simulink model "mpc_model_control_robot_with_forces"  (Simulink 8.0)
settings: Solver=ode3  StartTime=0.0  StopTime=delta_t  FixedStep=0.0002  RelTol=1e-3
values from neighbouring files (symbols this model uses):
  all_J_T_K_J = all_J_T_K_J + J_cont'*K_cont*J_cont    [run_control_tests_no_obstacles_testing_model_prediction.m]    (also in run_control_tests_with_force.m; run_control_tests_with_force_and_model_prediction.m; run_control_tests_with_force_kreacher.m; run_control_tests_with_force_vary_stiffness_and_delta_t.m)
  all_J_T_Kd_J = all_J_T_Kd_J + J_cont'*Kd_cont*J_cont    [run_control_tests_no_obstacles_testing_model_prediction.m]    (also in run_control_tests_with_force.m; run_control_tests_with_force_and_model_prediction.m; run_control_tests_with_force_vary_stiffness_and_delta_t.m; run_control_tests_with_obstacles_testing_model_prediction.m)
  Kd = diag([kd, kd, kd, kd])    [run_control_tests_no_force_vary_time_horizon_kreacher.m]    (also in run_control_tests_no_force_vary_time_horizon_kreacher_QS.m; run_control_tests_no_force_vary_time_horizon_single_link.m = diag([kd]); run_control_tests_no_force_vary_time_horizon_single_link_QS.m = diag([kd]); run_control_tests_no_obstacles_testing_model_prediction.m = diag([20, 15, 8]))
  Kp = diag([kp_vec(ll), kp_vec(ll), kp_vec(ll), kp_vec(ll)])    [run_control_tests_no_force_vary_time_horizon_kreacher.m]    (also in run_control_tests_no_force_vary_time_horizon_kreacher_QS.m; run_control_tests_no_force_vary_time_horizon_single_link.m = diag([kp_vec(ll)]); run_control_tests_no_force_vary_time_horizon_single_link_QS.m = diag([kp_vec(ll)]); run_control_tests_no_obstacles_testing_model_prediction.m = diag([30, 20, 15]))
  q_0 = q(end,:)    [run_control_tests_no_force_vary_time_horizon_kreacher.m]    (also in run_control_tests_no_force_vary_time_horizon_kreacher_QS.m; run_control_tests_no_force_vary_time_horizon_single_link.m; run_control_tests_no_force_vary_time_horizon_single_link_QS.m; run_control_tests_no_obstacles_testing_model_prediction.m)
  q_des = q_des_cur_0    [run_control_tests_no_force_vary_time_horizon_kreacher.m]    (also in run_control_tests_no_force_vary_time_horizon_kreacher_QS.m; run_control_tests_no_force_vary_time_horizon_single_link.m; run_control_tests_no_force_vary_time_horizon_single_link_QS.m; run_control_tests_no_obstacles_testing_model_prediction.m = q_des + vars.u_4')
  q_init = q_0    [run_control_tests_no_force_vary_time_horizon_kreacher.m]    (also in run_control_tests_no_force_vary_time_horizon_kreacher_QS.m; run_control_tests_no_force_vary_time_horizon_single_link.m; run_control_tests_no_force_vary_time_horizon_single_link_QS.m; run_control_tests_no_obstacles_testing_model_prediction.m = q_5(end,:))
  qd_init = qd_0    [run_control_tests_no_force_vary_time_horizon_kreacher.m]    (also in run_control_tests_no_force_vary_time_horizon_kreacher_QS.m; run_control_tests_no_force_vary_time_horizon_single_link.m; run_control_tests_no_force_vary_time_horizon_single_link_QS.m; run_control_tests_no_obstacles_testing_model_prediction.m = qd_5(end,:))
  tau_cont_sum_0 = tau_cont_sum_0 + J_cont'*f_vec    [run_control_tests_no_obstacles_testing_model_prediction.m]    (also in run_control_tests_with_force.m; run_control_tests_with_force_and_model_prediction.m; run_control_tests_with_force_kreacher.m; run_control_tests_with_force_vary_stiffness_and_delta_t.m)
undefined symbols (not defined in the file): robot
settings Model: Creator=pic  LastModifiedBy=mkillpack  ExtModeTrigMode=oneshot  ExtModeArmWhenConnect=off
settings DataIOCC: LimitDataPoints=off  SignalLoggingSaveFormat=ModelDataLogs  SignalLogging=off  ReturnWorkspaceOutputs=on
settings OptimizationCC: BlockReduction=off  BooleanDataType=off  InitFltsAndDblsToZero=on
settings DebuggingCC: SaveWithParameterizedLinksMsg=none  SignalResolutionControl=TryResolveAllWithWarning  SolverPrmCheckMsg=none  MultiTaskDSMMsg=warning  MultiTaskCondExecSysMsg=none  FcnCallInpInsideContextMsg=EnableAllAsWarning  StrictBusMsg=None
settings HardwareCC: TargetUnknown=on
settings RTWCC: IncludeERTFirstTime=on
settings GRTTargetCC: ModelReferenceCompliant=off  ParMdlRefBuildCompliant=off  CompOptLevelCompliant=off  CombineOutputUpdateFcns=off  MatFileLogging=off  GRTInterface=on

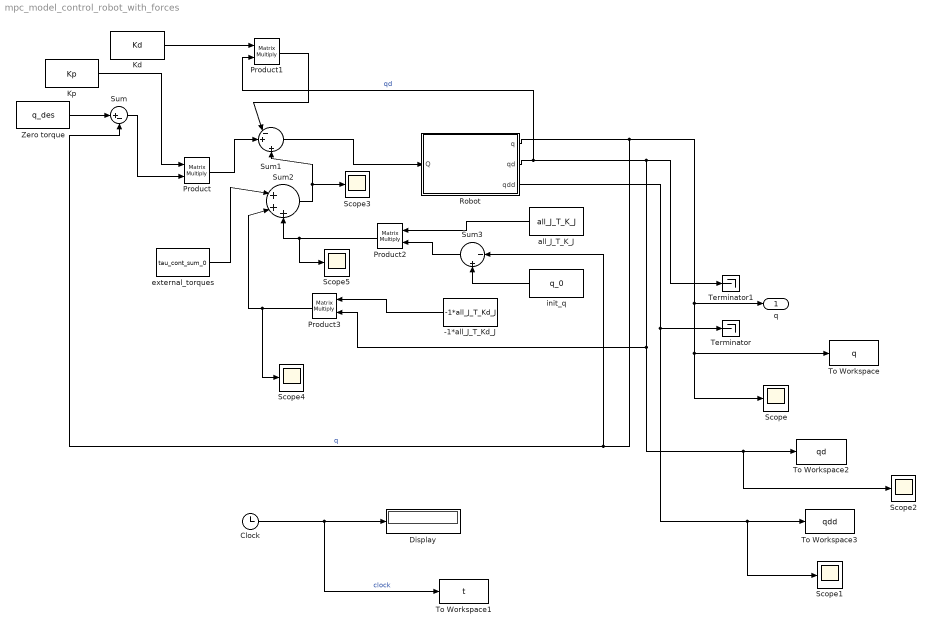
== system mpc_model_control_robot_with_forces ==
  -1*all_J_T_Kd_J : Constant  Value=-1*all_J_T_Kd_J
  Clock : Clock
  Display : Display
  Kd : Constant  Value=Kd
  Kp : Constant  Value=Kp
  Product{,1..3} (4 alike) : Product  Multiplication=Matrix(*)  RndMeth=Zero
  Robot : Subsystem  mask{robot=robot, q0=q_init}
      mask prompts: robot "Robot object"; q0 "Initial state"
      mask help: Rigid-body dynamic model of robot.
      mask init:
      | if isa(robot, 'SerialLink')
      |     rname = robot.name;
      |     %fprintf('**robot name is %s\n', rname);
      | else
      |     rname = '';
      |     n = 0
      | end
      mask Help:
      | Simulates the forward (direct) rigid-body dynamics of the robot described
      | by the given robot object.  For given applied joint torque/force it computes
      | the instaneous joint coordinates, velocities and acclerations.
      | 
      | 
      | <b>Parameters::</b>
      | 
      | robot (SerialLink) a dynamic model of an N-link serial link manipulator
      | q0 (1xN)  Initial joint coordinates
      | 
      | <b>Inputs::</b>
      | 
      | Q (1xN) the generalized joint force (torque or force) required to achieve
      | the motion state (q, qd, qdd).
      | 
      | <b>Outputs::</b>
      | 
      | q (1xN) joint coordinates
      | qd (1xN) joint coordinate velocity
      | qdd (1xN) joint coordinate acceleration
      | 
      | 
      | <b>Notes::</b>
      | 
      | - Required to simulate robot rigid body motion.
      | - Implemented using the recursive Newton-Euler scheme (RNE).
      | - A wrapper for the Toolbox method accel() which in turn depends on the
      |   method rne().
      mask Display:
      | port_label('input', 1, 'Q')
      | port_label('output', 1, 'q')
      | port_label('output', 2, 'qd')
      | port_label('output', 3, 'qdd')
      | text(0.1, 0.9,  rname, 'horizontalAlignment', 'left')
  Scope{,1..5} (6 alike) : Scope
      Scope settings: YMin=0.008275  YMax=0.00885
      Scope1 settings: YMin=-0.5  YMax=3.75
      Scope2 settings: YMin=0.008  YMax=0.0145  SaveName=ScopeData2
      Scope3 settings: YMin=0.008  YMax=0.0145  SaveName=ScopeData3
      Scope4 settings: YMin=0.008  YMax=0.0145  SaveName=ScopeData4
      Scope5 settings: YMin=0.008  YMax=0.0145  SaveName=ScopeData5
  Sum : Sum  Inputs=|+-
  Sum1 : Sum  Inputs=|-+|+
  Sum2 : Sum  Inputs=||+|+|+
  Sum3 : Sum  Inputs=||-|+
  Terminator : Terminator
  Terminator1 : Terminator
  To Workspace : ToWorkspace  VariableName=q  SampleTime=-1
  To Workspace1 : ToWorkspace  VariableName=t  SampleTime=-1
  To Workspace2 : ToWorkspace  VariableName=qd  SampleTime=-1
  To Workspace3 : ToWorkspace  VariableName=qdd  SampleTime=-1
  Zero torque : Constant  Value=q_des
  all_J_T_K_J : Constant  Value=all_J_T_K_J
  external_torques : Constant  Value=tau_cont_sum_0
  "init_q " : Constant  Value=q_0
  q : Outport
  wires:
  Robot/1(q) -> Scope/1, To Workspace/1, q/1, Sum/2, Sum3/1  "q"
  Robot/3(qdd) -> To Workspace3/1, Scope1/1, Terminator/1
  Robot/2(qd) -> Terminator1/1, To Workspace2/1, Scope2/1, Product3/2, Product1/2  "qd"
  Zero torque/1 -> Sum/1
  Sum/1 -> Product/2
  Sum1/1 -> Robot/1(Q)
  Clock/1 -> Display/1, To Workspace1/1  "clock"
  Kp/1 -> Product/1
  Product/1 -> Sum1/2
  Product1/1 -> Sum1/1
  Kd/1 -> Product1/1
  external_torques/1 -> Sum2/1
  "init_q "/1 -> Sum3/2
  Sum2/1 -> Scope3/1, Sum1/3
  Product2/1 -> Scope5/1, Sum2/3
  all_J_T_K_J/1 -> Product2/1
  -1*all_J_T_Kd_J/1 -> Product3/1
  Product3/1 -> Scope4/1, Sum2/2
  Sum3/1 -> Product2/2

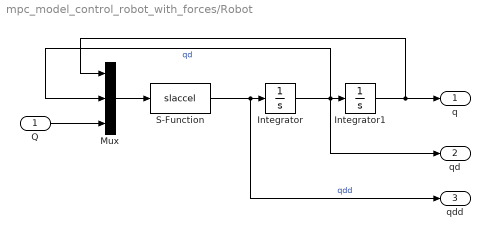
== system mpc_model_control_robot_with_forces/Robot ==
  Q : Inport
  Integrator : Integrator  InitialCondition=qd_init
  Integrator1 : Integrator  InitialCondition=q_init
  Mux : Mux  Inputs=3
  S-Function : S-Function  FunctionName=slaccel  Parameters=robot  EnableBusSupport=off
  q : Outport
  qd : Outport  Port=2
  qdd : Outport  Port=3
  wires:
  S-Function/1 -> qdd/1, Integrator/1  "qdd"
  Mux/1 -> S-Function/1
  Integrator/1 -> qd/1, Integrator1/1, Mux/2  "qd"
  Q/1 -> Mux/3
  Integrator1/1 -> q/1, Mux/1
